simulink model "gm_Approximate_id_46f54147700b843c92a4e9dfa9c6267fbdad2df7"  (R2020a)
settings: Solver=VariableStepAuto  StartTime=0.0  StopTime=10.0  RelTol=1e-3
model workspace (MAT data in the model file):
  InputValues_20210723T014030585 = [-8 -7.99975585938 -7.99951171875 -7.99926757812 -7.9990234375 -7.99877929688 -7.99853515625 -7.99829101562 -7.998046875 -7.99780273438 -7.99755859375 -7.99731445312 ... (65536 elements, 65536x1)]
(part 1 of 2)
settings Model: Creator=Mahsa  LastModifiedBy=Mahsa
settings OptimizationCC: BlockReduction=off  ConditionallyExecuteInputs=off
settings DebuggingCC: InheritedTsInSrcMsg=none

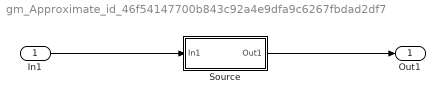
== system gm_Approximate_id_46f54147700b843c92a4e9dfa9c6267fbdad2df7 ==
  In1 : Inport  OutDataTypeStr=fixdt(1, 16, 12)  PortDimensions=1  SampleTime=0
  Source : Subsystem
  Out1 : Outport
  wires:
  In1/1 -> Source/1(In1)
  Source/1(Out1) -> Out1/1
